simulink model "c5mimp"  (R2022a)
settings: Solver=VariableStepAuto  StartTime=0.0  StopTime=10.0  RelTol=1e-3
undefined symbols (not defined in the file): N, nu, tau, ww
settings Model: Creator=xuedi  LastModifiedBy=xuedi

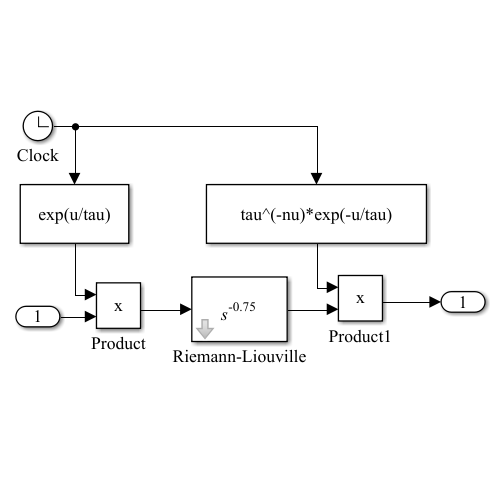
[thumbnail: Simulink's stored preview of the top-level diagram]
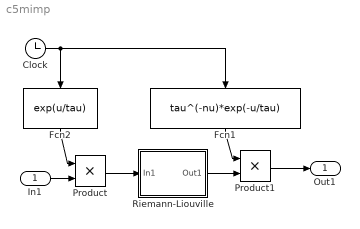
== system c5mimp ==
  In1 : Inport
  Clock : Clock
  Fcn1 : Fcn  Expr=tau^(-nu)*exp(-u/tau)
  Fcn2 : Fcn  Expr=exp(u/tau)
  Product : Product
  Product1 : Product
  "Riemann-Liouville " : Subsystem  mask{gam=-0.75, ww=ww, n=N, kF1=on, kF=Oustaloup filter}
      mask prompts: gam "Derivative order gamma"; ww "Frequency range [wb,wh]"; n "Apprixmation order"; kF1 "Is a low-pass filter required?"; kF "Filter type"
      mask init:
      | wb=ww(1); wh=ww(2); 
      | if kF==1, G=ousta_fod(gam,n,wb,wh);
      | else, G=new_fod(gam,n,wb,wh); end
      | G=tf(G); num=G.num{1}; den=G.den{1}; T=1/wh; 
      | if isnumeric(gam), str=['{\its}^{' num2str(gam) '}']; 
      | else, str='{\its}^{gam}'; end
      | if kF1==1, G=G*tf(1,[T 1]); end
      mask TypeOptions kF: Oustaloup filter | Modified Oustaloup filter | Matsuda-Fujii filter
      mask Display: disp(str,'texmode','on')
  Out1 : Outport
  wires:
  "Riemann-Liouville "/1(Out1) -> Product1/2
  Fcn1/1 -> Product1/1
  In1/1 -> Product/2
  Fcn2/1 -> Product/1
  Clock/1 -> Fcn2/1, Fcn1/1
  Product1/1 -> Out1/1
  Product/1 -> "Riemann-Liouville "/1(In1)

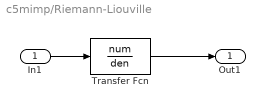
== system c5mimp/Riemann-Liouville  ==
  In1 : Inport
  Transfer Fcn : TransferFcn  Numerator=num  Denominator=den
  Out1 : Outport
  wires:
  Transfer Fcn/1 -> Out1/1
  In1/1 -> Transfer Fcn/1
